simulink model "PID_3R_2020a"  (R2020a)
settings: Solver=VariableStepAuto  StartTime=0.0  StopTime=10  RelTol=1e-3
libraries: simulink x3
settings Model: Creator=Javad  LastModifiedBy=Alireza

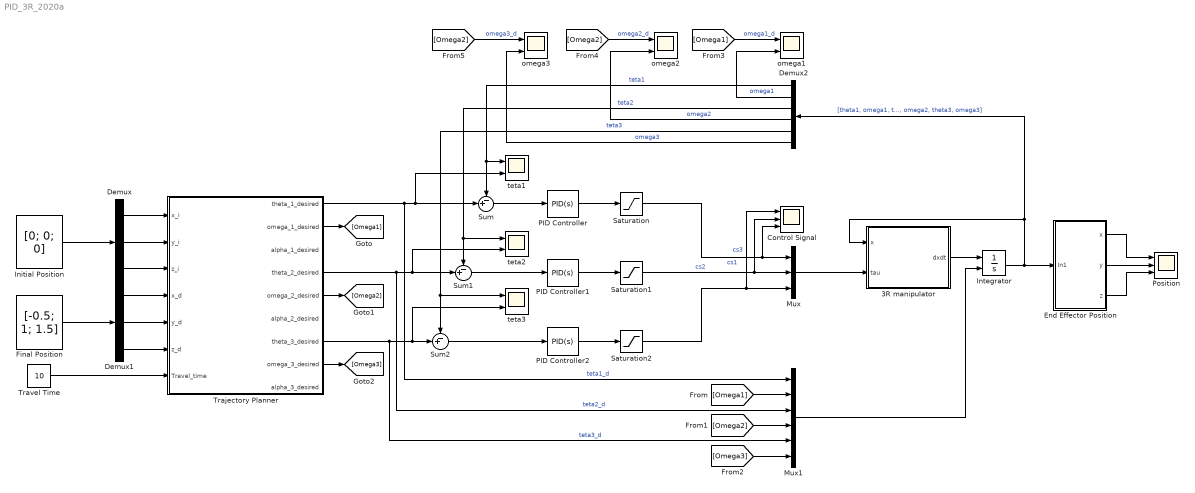
== system PID_3R_2020a ==
  3R manipulator : MATLAB Function  TreatAsAtomicUnit=on
  Control Signal : Scope  NumInputPorts=3
  Demux : Demux  Outputs=3
  Demux1 : Demux  Outputs=3
  Demux2 : Demux  Outputs=6
  End Effector Position : Subsystem
  Final Position : Constant  Value=[-0.5; 1; 1.5]  VectorParams1D=off
  Initial Position : Constant  Value=[0; 0; 0]  VectorParams1D=off
  Integrator : Integrator  InitialConditionSource=external
  Mux : Mux  Inputs=3
  Mux1 : Mux  Inputs=6
  PID Controller : simulink/Continuous/PID Controller  Controller=PID  Form=Parallel  TimeDomain=Continuous-time  UseExternalTs=off  SampleTime=-1  IntegratorMethod=Forward Euler  FilterMethod=Forward Euler  ControllerParametersSource=internal  P=2.75  I=0.16  D=10.5  UseFilter=on  N=1100  TunerSelectOption=Transfer Function Based (PID Tuner App)  InitialConditionSource=internal  InitialConditionForIntegrator=0  InitialConditionForFilter=0  DifferentiatorICPrevScaledInput=0  ExternalReset=none  TrackingMode=off  Kt=1  LimitOutput=off  UpperSaturationLimit=inf  LowerSaturationLimit=-inf  LinearizeAsGain=on  AntiWindupMode=none  Kb=1  POutMin=[]  POutMax=[]  IOutMin=[]  IOutMax=[]  DOutMin=[]  DOutMax=[]  NOutMin=[]  NOutMax=[]  SumOutMin=[]  SumOutMax=[]  SaturationOutMin=[]  SaturationOutMax=[]  PParamMin=[]  PParamMax=[]  IParamMin=[]  IParamMax=[]  DParamMin=[]  DParamMax=[]  NParamMin=[]  NParamMax=[]  KbParamMin=[]  KbParamMax=[]  KtParamMin=[]  KtParamMax=[]  KbOutMin=[]  KbOutMax=[]  KtOutMin=[]  KtOutMax=[]  IntegratorOutMin=[]  IntegratorOutMax=[]  FilterOutMin=[]  FilterOutMax=[]  SumI1OutMin=[]  SumI1OutMax=[]  SumI2OutMin=[]  SumI2OutMax=[]  SumI3OutMin=[]  SumI3OutMax=[]  SumI4OutMin=[]  SumI4OutMax=[]  SumDOutMin=[]  SumDOutMax=[]  DifferentiatorOutMin=[]  DifferentiatorOutMax=[]  FilterDiffOutCoefMin=[]  FilterDiffOutCoefMax=[]  ReciprocalOutMin=[]  ReciprocalOutMax=[]  SumDenOutMin=[]  SumDenOutMax=[]  SumNumOutMin=[]  SumNumOutMax=[]  DivideOutMin=[]  DivideOutMax=[]  UdiffTsProdOutMin=[]  UdiffTsProdOutMax=[]  NTsProdOutMin=[]  NTsProdOutMax=[]  UintegralTsProdOutMin=[]  UintegralTsProdOutMax=[]  UngainTsProdOutMin=[]  UngainTsProdOutMax=[]  IntegratorContinuousStateAttributes=''  IntegratorStateMustResolveToSignalObject=off  IntegratorRTWStateStorageClass=Auto  FilterContinuousStateAttributes=''  FilterStateMustResolveToSignalObject=off  FilterRTWStateStorageClass=Auto  ParallelPVariant=InternalParameters  IdealPVariant=Disabled  IVariant=InternalParameters  DVariant=InternalParameters  IntegratorVariant=Continuous  SatVariant=Disabled  AWVariant=Passthrough  PCopyVariant=Disabled  TRVariant=Disabled  FdbkBlocksVariant=Forward  IdealPFdbkVariant=Disabled  SatFdbkVariant=Disabled  DerivativeFilterVariant=ContFilter  NVariant=InternalParameters  NCopyVariant=Disabled  FilterICVariant=InternalICsFilter  IntegratorICVariant=InternalICs  ExternalResetVariant=Disabled  TRSumVariant=Passthrough  SumFdbkVariant=Disabled  SumVariant=Sum_PID  TsampFilterVariant=InternalTs  TsampNgainVariant=Passthrough  TsampIntegralVariant=Passthrough
  PID Controller1 : simulink/Continuous/PID Controller  Controller=PID  Form=Parallel  TimeDomain=Continuous-time  UseExternalTs=off  SampleTime=-1  IntegratorMethod=Forward Euler  FilterMethod=Forward Euler  ControllerParametersSource=internal  P=1200  I=2500  D=250  UseFilter=on  N=1100  TunerSelectOption=Transfer Function Based (PID Tuner App)  InitialConditionSource=internal  InitialConditionForIntegrator=0  InitialConditionForFilter=0  DifferentiatorICPrevScaledInput=0  ExternalReset=none  TrackingMode=off  Kt=1  LimitOutput=off  UpperSaturationLimit=inf  LowerSaturationLimit=-inf  LinearizeAsGain=on  AntiWindupMode=none  Kb=1  POutMin=[]  POutMax=[]  IOutMin=[]  IOutMax=[]  DOutMin=[]  DOutMax=[]  NOutMin=[]  NOutMax=[]  SumOutMin=[]  SumOutMax=[]  SaturationOutMin=[]  SaturationOutMax=[]  PParamMin=[]  PParamMax=[]  IParamMin=[]  IParamMax=[]  DParamMin=[]  DParamMax=[]  NParamMin=[]  NParamMax=[]  KbParamMin=[]  KbParamMax=[]  KtParamMin=[]  KtParamMax=[]  KbOutMin=[]  KbOutMax=[]  KtOutMin=[]  KtOutMax=[]  IntegratorOutMin=[]  IntegratorOutMax=[]  FilterOutMin=[]  FilterOutMax=[]  SumI1OutMin=[]  SumI1OutMax=[]  SumI2OutMin=[]  SumI2OutMax=[]  SumI3OutMin=[]  SumI3OutMax=[]  SumI4OutMin=[]  SumI4OutMax=[]  SumDOutMin=[]  SumDOutMax=[]  DifferentiatorOutMin=[]  DifferentiatorOutMax=[]  FilterDiffOutCoefMin=[]  FilterDiffOutCoefMax=[]  ReciprocalOutMin=[]  ReciprocalOutMax=[]  SumDenOutMin=[]  SumDenOutMax=[]  SumNumOutMin=[]  SumNumOutMax=[]  DivideOutMin=[]  DivideOutMax=[]  UdiffTsProdOutMin=[]  UdiffTsProdOutMax=[]  NTsProdOutMin=[]  NTsProdOutMax=[]  UintegralTsProdOutMin=[]  UintegralTsProdOutMax=[]  UngainTsProdOutMin=[]  UngainTsProdOutMax=[]  IntegratorContinuousStateAttributes=''  IntegratorStateMustResolveToSignalObject=off  IntegratorRTWStateStorageClass=Auto  FilterContinuousStateAttributes=''  FilterStateMustResolveToSignalObject=off  FilterRTWStateStorageClass=Auto  ParallelPVariant=InternalParameters  IdealPVariant=Disabled  IVariant=InternalParameters  DVariant=InternalParameters  IntegratorVariant=Continuous  SatVariant=Disabled  AWVariant=Passthrough  PCopyVariant=Disabled  TRVariant=Disabled  FdbkBlocksVariant=Forward  IdealPFdbkVariant=Disabled  SatFdbkVariant=Disabled  DerivativeFilterVariant=ContFilter  NVariant=InternalParameters  NCopyVariant=Disabled  FilterICVariant=InternalICsFilter  IntegratorICVariant=InternalICs  ExternalResetVariant=Disabled  TRSumVariant=Passthrough  SumFdbkVariant=Disabled  SumVariant=Sum_PID  TsampFilterVariant=InternalTs  TsampNgainVariant=Passthrough  TsampIntegralVariant=Passthrough
  PID Controller2 : simulink/Continuous/PID Controller  Controller=PID  Form=Parallel  TimeDomain=Continuous-time  UseExternalTs=off  SampleTime=-1  IntegratorMethod=Forward Euler  FilterMethod=Forward Euler  ControllerParametersSource=internal  P=174  I=325  D=78.5  UseFilter=on  N=1100  TunerSelectOption=Transfer Function Based (PID Tuner App)  InitialConditionSource=internal  InitialConditionForIntegrator=0  InitialConditionForFilter=0  DifferentiatorICPrevScaledInput=0  ExternalReset=none  TrackingMode=off  Kt=1  LimitOutput=off  UpperSaturationLimit=inf  LowerSaturationLimit=-inf  LinearizeAsGain=on  AntiWindupMode=none  Kb=1  POutMin=[]  POutMax=[]  IOutMin=[]  IOutMax=[]  DOutMin=[]  DOutMax=[]  NOutMin=[]  NOutMax=[]  SumOutMin=[]  SumOutMax=[]  SaturationOutMin=[]  SaturationOutMax=[]  PParamMin=[]  PParamMax=[]  IParamMin=[]  IParamMax=[]  DParamMin=[]  DParamMax=[]  NParamMin=[]  NParamMax=[]  KbParamMin=[]  KbParamMax=[]  KtParamMin=[]  KtParamMax=[]  KbOutMin=[]  KbOutMax=[]  KtOutMin=[]  KtOutMax=[]  IntegratorOutMin=[]  IntegratorOutMax=[]  FilterOutMin=[]  FilterOutMax=[]  SumI1OutMin=[]  SumI1OutMax=[]  SumI2OutMin=[]  SumI2OutMax=[]  SumI3OutMin=[]  SumI3OutMax=[]  SumI4OutMin=[]  SumI4OutMax=[]  SumDOutMin=[]  SumDOutMax=[]  DifferentiatorOutMin=[]  DifferentiatorOutMax=[]  FilterDiffOutCoefMin=[]  FilterDiffOutCoefMax=[]  ReciprocalOutMin=[]  ReciprocalOutMax=[]  SumDenOutMin=[]  SumDenOutMax=[]  SumNumOutMin=[]  SumNumOutMax=[]  DivideOutMin=[]  DivideOutMax=[]  UdiffTsProdOutMin=[]  UdiffTsProdOutMax=[]  NTsProdOutMin=[]  NTsProdOutMax=[]  UintegralTsProdOutMin=[]  UintegralTsProdOutMax=[]  UngainTsProdOutMin=[]  UngainTsProdOutMax=[]  IntegratorContinuousStateAttributes=''  IntegratorStateMustResolveToSignalObject=off  IntegratorRTWStateStorageClass=Auto  FilterContinuousStateAttributes=''  FilterStateMustResolveToSignalObject=off  FilterRTWStateStorageClass=Auto  ParallelPVariant=InternalParameters  IdealPVariant=Disabled  IVariant=InternalParameters  DVariant=InternalParameters  IntegratorVariant=Continuous  SatVariant=Disabled  AWVariant=Passthrough  PCopyVariant=Disabled  TRVariant=Disabled  FdbkBlocksVariant=Forward  IdealPFdbkVariant=Disabled  SatFdbkVariant=Disabled  DerivativeFilterVariant=ContFilter  NVariant=InternalParameters  NCopyVariant=Disabled  FilterICVariant=InternalICsFilter  IntegratorICVariant=InternalICs  ExternalResetVariant=Disabled  TRSumVariant=Passthrough  SumFdbkVariant=Disabled  SumVariant=Sum_PID  TsampFilterVariant=InternalTs  TsampNgainVariant=Passthrough  TsampIntegralVariant=Passthrough
  Position : Scope  NumInputPorts=3
  Saturation : Saturate  UpperLimit=15  LowerLimit=-15
  Saturation1 : Saturate  UpperLimit=15  LowerLimit=-15
  Saturation2 : Saturate  UpperLimit=15  LowerLimit=-15
  Sum : Sum  Inputs=-+|
  Sum1 : Sum  Inputs=-+|
  Sum2 : Sum  Inputs=-+|
  Trajectory Planner : Subsystem
  "Travel Time " : Constant  Value=10
  omega1 : Scope  NumInputPorts=2
  omega2 : Scope  NumInputPorts=2
  omega3 : Scope  NumInputPorts=2
  teta1 : Scope  NumInputPorts=2
  teta2 : Scope  NumInputPorts=2
  teta3 : Scope  NumInputPorts=2
  wires:
  3R manipulator/1(dxdt) -> Integrator/1
  Integrator/1 -> Demux2/1, 3R manipulator/1(x), End Effector Position/1(In1)  "[theta1, omega1, theta2, omega2, theta3, omega3]"
  Demux2/5 -> teta3/1, Sum2/1  "teta3"
  Saturation2/1 -> Control Signal/1, Mux/3  "cs3"
  Mux/1 -> 3R manipulator/2(tau)
  Demux2/1 -> teta1/1, Sum/1  "teta1"
  Sum2/1 -> PID Controller2/1
  End Effector Position/1(x) -> Position/1
  End Effector Position/2(y) -> Position/2
  End Effector Position/3(z) -> Position/3
  Saturation1/1 -> Control Signal/2, Mux/2  "cs2"
  Sum1/1 -> PID Controller1/1
  Saturation/1 -> Control Signal/3, Mux/1  "cs1"
  Sum/1 -> PID Controller/1
  Trajectory Planner/1(theta_1_desired) -> teta1/2, Sum/2, Mux1/1  "teta1_d"
  Trajectory Planner/4(theta_2_desired) -> teta2/2, Sum1/2, Mux1/3  "teta2_d"
  Trajectory Planner/7(theta_3_desired) -> teta3/2, Sum2/2, Mux1/5  "teta3_d"
  Demux2/3 -> teta2/1, Sum1/1  "teta2"
  Final Position/1 -> Demux1/1
  Demux1/2 -> Trajectory Planner/5(y_d)
  Demux/3 -> Trajectory Planner/3(z_i)
  "Travel Time "/1 -> Trajectory Planner/7(Travel_time)
  Demux1/3 -> Trajectory Planner/6(z_d)
  Demux1/1 -> Trajectory Planner/4(x_d)
  Demux/2 -> Trajectory Planner/2(y_i)
  Initial Position/1 -> Demux/1
  Demux/1 -> Trajectory Planner/1(x_i)
  Trajectory Planner/2(omega_1_desired) -> [Omega1]
  Trajectory Planner/5(omega_2_desired) -> [Omega2]
  Trajectory Planner/8(omega_3_desired) -> [Omega3]
  [Omega1] -> Mux1/2
  [Omega2] -> Mux1/4
  [Omega3] -> Mux1/6
  Mux1/1 -> Integrator/2
  [Omega1] -> omega1/1  "omega1_d"
  [Omega2] -> omega2/1  "omega2_d"
  [Omega2] -> omega3/1  "omega3_d"
  Demux2/2 -> omega1/2  "omega1"
  Demux2/4 -> omega2/2  "omega2"
  Demux2/6 -> omega3/2  "omega3"
  PID Controller/1 -> Saturation/1
  PID Controller1/1 -> Saturation1/1
  PID Controller2/1 -> Saturation2/1

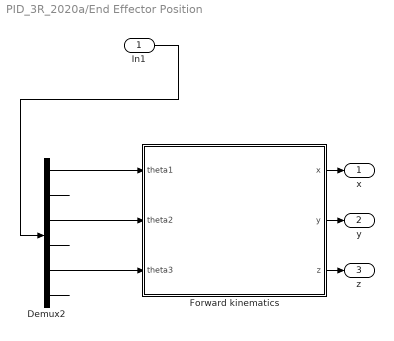
== system PID_3R_2020a/End Effector Position ==
  In1 : Inport
  Demux2 : Demux  Outputs=6
  Forward kinematics : MATLAB Function  TreatAsAtomicUnit=on
  x : Outport
  y : Outport  Port=2
  z : Outport  Port=3
  wires:
  Demux2/1 -> Forward kinematics/1(theta1)
  In1/1 -> Demux2/1
  Forward kinematics/2(y) -> y/1
  Demux2/3 -> Forward kinematics/2(theta2)
  Demux2/4 -> ?
  Forward kinematics/3(z) -> z/1
  Forward kinematics/1(x) -> x/1
  Demux2/2 -> ?
  Demux2/5 -> Forward kinematics/3(theta3)
  Demux2/6 -> ?

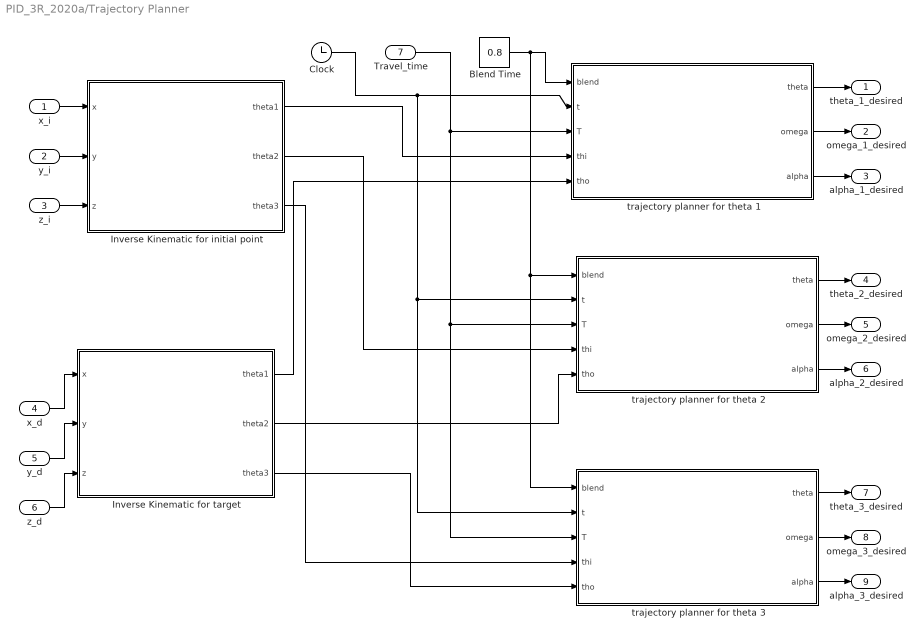
== system PID_3R_2020a/Trajectory Planner ==
  x_i : Inport
  y_i : Inport  Port=2
  z_i : Inport  Port=3
  x_d : Inport  Port=4
  y_d : Inport  Port=5
  z_d : Inport  Port=6
  Travel_time : Inport  Port=7
  Blend Time : Constant  Value=0.8
  Clock : Clock
  Inverse Kinematic for initial point : MATLAB Function  TreatAsAtomicUnit=on
  Inverse Kinematic for target : MATLAB Function  TreatAsAtomicUnit=on
  trajectory planner for theta 1 : MATLAB Function  TreatAsAtomicUnit=on
  trajectory planner for theta 2 : MATLAB Function  TreatAsAtomicUnit=on
  trajectory planner for theta 3 : MATLAB Function  TreatAsAtomicUnit=on
  theta_1_desired : Outport
  omega_1_desired : Outport  Port=2
  alpha_1_desired : Outport  Port=3
  theta_2_desired : Outport  Port=4
  omega_2_desired : Outport  Port=5
  alpha_2_desired : Outport  Port=6
  theta_3_desired : Outport  Port=7
  omega_3_desired : Outport  Port=8
  alpha_3_desired : Outport  Port=9
  wires:
  trajectory planner for theta 1/2(omega) -> omega_1_desired/1
  y_i/1 -> Inverse Kinematic for initial point/2(y)
  trajectory planner for theta 1/1(theta) -> theta_1_desired/1
  Inverse Kinematic for initial point/1(theta1) -> trajectory planner for theta 1/4(thi)
  Inverse Kinematic for target/1(theta1) -> trajectory planner for theta 1/5(tho)
  trajectory planner for theta 1/3(alpha) -> alpha_1_desired/1
  x_i/1 -> Inverse Kinematic for initial point/1(x)
  z_i/1 -> Inverse Kinematic for initial point/3(z)
  Inverse Kinematic for initial point/2(theta2) -> trajectory planner for theta 2/4(thi)
  trajectory planner for theta 2/3(alpha) -> alpha_2_desired/1
  trajectory planner for theta 2/2(omega) -> omega_2_desired/1
  trajectory planner for theta 2/1(theta) -> theta_2_desired/1
  Inverse Kinematic for target/2(theta2) -> trajectory planner for theta 2/5(tho)
  Clock/1 -> trajectory planner for theta 1/2(t), trajectory planner for theta 3/2(t), trajectory planner for theta 2/2(t)
  Inverse Kinematic for target/3(theta3) -> trajectory planner for theta 3/5(tho)
  trajectory planner for theta 3/1(theta) -> theta_3_desired/1
  Inverse Kinematic for initial point/3(theta3) -> trajectory planner for theta 3/4(thi)
  Travel_time/1 -> trajectory planner for theta 1/3(T), trajectory planner for theta 2/3(T), trajectory planner for theta 3/3(T)
  trajectory planner for theta 3/2(omega) -> omega_3_desired/1
  Blend Time/1 -> trajectory planner for theta 2/1(blend), trajectory planner for theta 3/1(blend), trajectory planner for theta 1/1(blend)
  trajectory planner for theta 3/3(alpha) -> alpha_3_desired/1
  z_d/1 -> Inverse Kinematic for target/3(z)
  x_d/1 -> Inverse Kinematic for target/1(x)
  y_d/1 -> Inverse Kinematic for target/2(y)

== matlab function PID_3R_2020a/Trajectory Planner/Inverse Kinematic for initial point ==
  data: x input; theta1 output; y input; z input; theta2 output; theta3 output
function [theta1, theta2, theta3] = inverse_kinematic(x, y, z)

L1=1.5; L2=0.8; L3=0.7;
theta1 = atan2(y, x);
theta3 = acos((x^2+y^2+(z-L1)^2-L2^2-L3^2)/(2*L2*L3));
phi = atan2(L3*sin(theta3), L3*cos(theta3)+L2);
disp(phi/pi*180)
theta2 = asin((z-L1)*cos(phi)/(L3*cos(theta3)+L2))-phi;

end

== matlab function PID_3R_2020a/3R manipulator ==
  data: x input size=[6,1]; dxdt output size=[6,1]; tau input size=[3,1]

function dxdt = Plant_3R (x, tau)
th1 = x(1);
th1_d = x(2);
th2 = x(3);
th2_d = x(4);
th3 = x(5);
th3_d = x(6);
dxdt = zeros(6,1);
dxdt(1) = th1_d;
dxdt(2) = (2.4e+3*tau(1)-670.0*th1_d*th2_d*sin(th3)+...
    290.0*th1_d*th2_d*sin(2.0*th2+2.0*th3)+...
    290.0*th1_d*th3_d*sin(2.0*th2+2.0*th3)+...
    670.0*th1_d*th2_d*sin(2.0*th2+th3)+...
    380.0*th1_d*th2_d*sin(2.0*th2))/(340.0*cos(2.0*th2+th3)+...
    190.0*cos(2.0*th2)+340.0*cos(th3)+150.0*cos(2.0*th2+2.0*th3)+1.5e+3);
dxdt(3) = th2_d;
dxdt(4) = -0.38*sin(2.0*th2)*th1_d^2-18.0*cos(th2)+4.7*tau(2)-4.7*tau(3);
dxdt(5) = th3_d;
dxdt(6) = 16.0*cos(th2-1.0*th3)+85.0*cos(th2+th3)+18.0*cos(th2)-...
    0.86*th1_d^2*sin(th3)-1.7*th2_d^2*sin(th3)+...
    0.32*th1_d^2*sin(2.0*th2-1.0*th3)-...
    0.38*th1_d^2*sin(2.0*th2+2.0*th3)-...
    0.54*th1_d^2*sin(2.0*th2+th3)+0.38*th1_d^2*sin(2.0*th2)+...
    11.0*tau(3)-4.7*tau(2);

end

== matlab function PID_3R_2020a/Trajectory Planner/trajectory planner for theta 1 ==
  data: blend input; t input; theta output; T input; thi input; tho input; omega output; alpha output
function [theta, omega, alpha] = trajectory_planner(blend, t, T, thi, tho)
%t is the current time
%T is the toal time of the movement. 
%thi is the initial angle
%tho is the target angle
% blend = 1;

V_max = (tho-thi)/(T-blend);
a = V_max/blend;

if t<=blend
    alpha = a;
    omega = a*t;
    theta = 1/2*a*t.^2+thi;
elseif t<=(T-blend)
    alpha = 0;
    omega = V_max;
    theta = 1/2*a*blend^2+thi+V_max.*(t-blend);
else
    alpha = -a;
    omega = V_max-a.*(t-(T-blend));
    theta = -1/2*a.*(t-(T-blend)).^2+V_max*(t-(T-blend))+1/2*a*blend^2+thi+...
        V_max*(T-2*blend);
end
    
end

== matlab function PID_3R_2020a/Trajectory Planner/trajectory planner for theta 2 ==
  data: blend input; t input; theta output; T input; thi input; tho input; omega output; alpha output
function [theta, omega, alpha] = trajectory_planner(blend, t, T, thi, tho)
%t is the current time
%T is the toal time of the movement. 
%thi is the initial angle
%tho is the target angle
blend = 1;

V_max = (tho-thi)/(T-blend);
a = V_max/blend;

if t<=blend
    alpha = a;
    omega = a*t;
    theta = 1/2*a*t.^2+thi;
elseif t<=(T-blend)
    alpha = 0;
    omega = V_max;
    theta = 1/2*a*blend^2+thi+V_max.*(t-blend);
else
    alpha = -a;
    omega = V_max-a.*(t-(T-blend));
    theta = -1/2*a.*(t-(T-blend)).^2+V_max*(t-(T-blend))+1/2*a*blend^2+thi+...
        V_max*(T-2*blend);
end
    
end

== matlab function PID_3R_2020a/Trajectory Planner/trajectory planner for theta 3 ==
  data: blend input; t input; theta output; T input; thi input; tho input; omega output; alpha output
function [theta, omega, alpha] = trajectory_planner(blend, t, T, thi, tho)
%t is the current time
%T is the toal time of the movement. 
%thi is the initial angle
%tho is the target angle
blend = 1;

V_max = (tho-thi)/(T-blend);
a = V_max/blend;

if t<=blend
    alpha = a;
    omega = a*t;
    theta = 1/2*a*t.^2+thi;
elseif t<=(T-blend)
    alpha = 0;
    omega = V_max;
    theta = 1/2*a*blend^2+thi+V_max.*(t-blend);
else
    alpha = -a;
    omega = V_max-a.*(t-(T-blend));
    theta = -1/2*a.*(t-(T-blend)).^2+V_max*(t-(T-blend))+1/2*a*blend^2+thi+...
        V_max*(T-2*blend);
end
    
end

== matlab function PID_3R_2020a/Trajectory Planner/Inverse Kinematic for target ==
  data: x input; theta1 output; y input; z input; theta2 output; theta3 output
function [theta1, theta2, theta3] = inverse_kinematic(x, y, z)

L1=1.5; L2=0.8; L3=0.7;
theta1 = atan2(y, x);
theta3 = acos((x^2+y^2+(z-L1)^2-L2^2-L3^2)/(2*L2*L3));
phi = atan2(L3*sin(theta3), L3*cos(theta3)+L2);
disp(phi/pi*180)
theta2 = asin((z-L1)*cos(phi)/(L3*cos(theta3)+L2))-phi;

end

== matlab function PID_3R_2020a/End Effector Position/Forward kinematics ==
  data: x output; theta1 input; y output; theta2 input; theta3 input; z output
function [x, y, z] = fcn(theta1, theta2, theta3)
L1=1.5; L2=0.8; L3=0.7;T_01 = [cos(theta1) -sin(theta1) 0  0;
        sin(theta1)  cos(theta1) 0  0;
        0            0           1  0;
        0            0           0  1];
    
T_12 = [cos(theta2) -sin(theta2) 0  0;
        0            0          -1  0;
        sin(theta2)  cos(theta2) 0  0;
        0            0           0  1];
    
T_23 = [cos(theta3) -sin(theta3) 0  L2;
        sin(theta3)  cos(theta3) 0  0;
        0            0           1  0;
        0            0           0  1];

T_34 = [1            0           0  L3;
        0            1           0  0;
        0            0           1  0;
        0            0           0  1];
    
T_04 = (T_01*T_12*T_23*T_34);

x = T_04(1,4);
y = T_04(2,4);
z = T_04(3,4)+L1;
end
